simulink model "RailP_DD1ms"  (R2016b)
settings: configuration reference "CodeGenConfigSet" (kept outside this file)
settings Model: Creator=lenovo  LastModifiedBy=zhoutinglin
settings ConfigSetRef: SourceLocation=Base Workspace

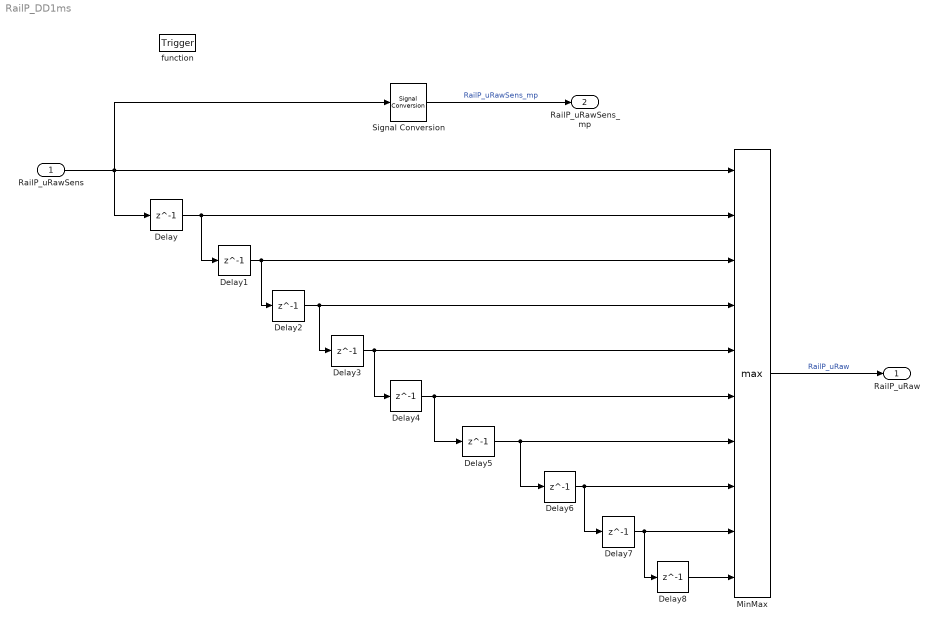
== system RailP_DD1ms ==
  RailP_uRawSens : Inport  Tag=mv  Description=Raw value of rail pressure  OutMin=0  OutMax=5000  OutDataTypeStr=Ad_mv
  function : TriggerPort  TriggerType=function-call  VariantControl=Variant
  Delay{,1..8} (9 alike) : Delay  DelayLength=1  InitialCondition=0
  MinMax : MinMax  Function=max  Inputs=10  InputSameDT=on
  Signal Conversion : SignalConversion  OverrideOpt=off
  RailP_uRaw : Outport  Tag=mv  Description=Raw value of rail pressure  OutMin=0  OutMax=5000  OutDataTypeStr=Ad_mv
  RailP_uRawSens_mp : Outport  Tag=mv  Description=Raw value of rail pressure before Peak Selection  Port=2  OutMin=0  OutMax=5000  OutDataTypeStr=Ad_mv
  wires:
  MinMax/1 -> RailP_uRaw/1  "RailP_uRaw"
  Delay2/1 -> MinMax/4, Delay3/1
  Delay3/1 -> MinMax/5, Delay4/1
  Delay4/1 -> MinMax/6, Delay5/1
  Delay5/1 -> MinMax/7, Delay6/1
  Delay6/1 -> MinMax/8, Delay7/1
  Delay7/1 -> MinMax/9, Delay8/1
  Delay8/1 -> MinMax/10
  Delay1/1 -> MinMax/3, Delay2/1
  Delay/1 -> MinMax/2, Delay1/1
  RailP_uRawSens/1 -> Signal Conversion/1, MinMax/1, Delay/1
  Signal Conversion/1 -> RailP_uRawSens_mp/1  "RailP_uRawSens_mp"
